simulink model "three_phase_pump"  (R2018a)
settings: Solver=VariableStepDiscrete  StartTime=0.0  StopTime=3  RelTol=1e-3
values from neighbouring files (symbols this model uses):
  Ts = 0.0001    [pump_ori_perf.mat]
libraries: fl_lib x8, sh_lib x5, nesl_utility x5, powerlib x2, electricdrivelib x1, powerlib_meascontrol x1
settings Model: Creator=siwak  LastModifiedBy=siwak

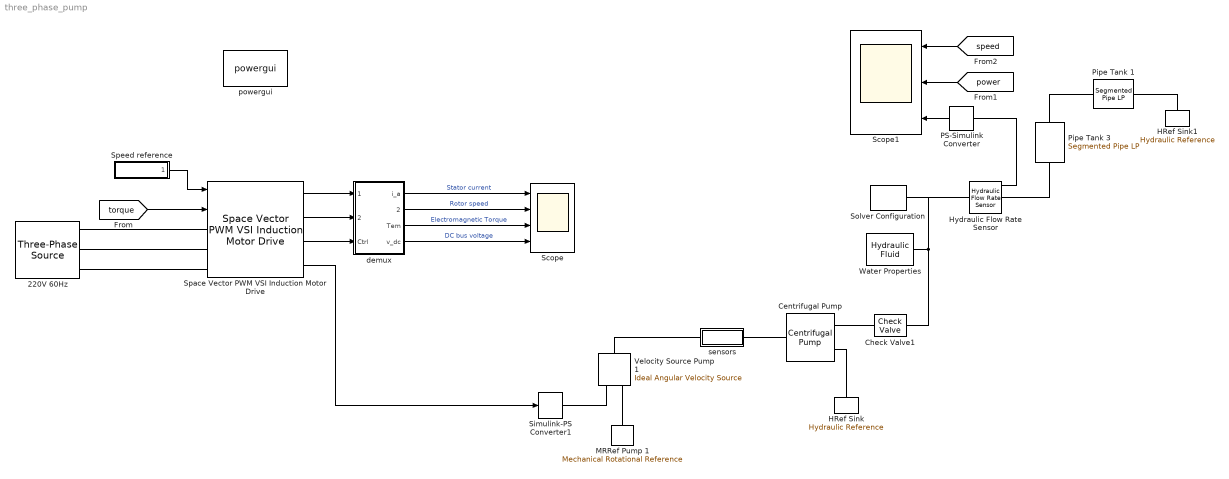
== system three_phase_pump ==
  220V 60Hz : powerlib/Electrical Sources/Three-Phase Source  InternalConnection=Yg  VoltagePhases=off  Voltage=220  PhaseAngle=0  Voltage_phases=[25e3 25e3 25e3]/sqrt(3)  PhaseAngles_phases=[0 -120 +120]  Frequency=60  NonIdealSource=on  SpecifyImpedance=off  Resistance=0.02  Inductance=0.05e-3  ShortCircuitLevel=100e6  BaseVoltage=25e3  XRratio=7  BusType=swing  Pref=0  Qref=0  Prefabc=[10e3, 10e3, 10e3]  Qrefabc=[0, 0, 0]  Qmin=-inf  Qmax=inf
  Centrifugal Pump : sh_lib/Pumps and Motors/Centrifugal Pump  mdl_type=2  c_1=326.8 Pa/(kg/m^3)  c_2=3.104e+4 Pa*s/kg  c_3=1.097e+7 Pa*s^2/(kg*m^3)  c_4=2.136e+5 Pa*s^2/(kg*m^3)  c_f=0.8  design_del=130 lpm  ref_velocity=1.77e+3 rpm  ref_density=940 kg/m^3  leak_resistance=1e+8 Pa/(m^3/s)  T_const=0.1 N*m  trq_press_coeff=1e-6 N*m/Pa  pump_del_1D="[ 0  20.0   64.2   92.8  110.0  130.0] gpm"  press_diff_1D=[50.97 47.08 39.12 31.39 23.6 15.69] psi  pump_del_power_1D="[ 0  20.0   64.2   92.8  110.0  130.0] gpm"  power_1D="[0 7.8e-01   2.1   2.4   2.16   1.7] HP"  pump_vel_2D=[ 3.2e+3 3.3e+3 3.4e+3 3.5e+3 ] rpm  pump_del_2D=[ 0 50 100 150 200 250 300 350 ] lpm  press_diff_2D=[ 8.3 8.8 9.3 9.9; 7.8 8.3 8.8 9.4; 7.2 7.6 8.2 8.7; 6.5 7 7.5 8; 5.6 6.1 6.6 7.1; 4.7 5.2 5.7 6.2; 3.4 4 4.4 4.9; 2.3 2.7 3.4 3.6 ] bar  pump_del_power_2D=[ 0 50 100 150 200 250 300 350 ] lpm  power_2D=[ 1.223e+3 1.341e+3 1.467e+3 1.6e+3; 1.414e+3 1.551e+3 1.696e+3 1.85e+3; 1.636e+3 1.794e+3 1.962e+3 2.14e+3; 1.941e+3 2.129e+3 2.326e+3 2.54e+3; 2.224e+3 2.439e+3 2.66e+3 2.91e+3; 2.453e+3 2.691e+3 2.947e+3 3.21e+3; 2.757e+3 3.024e+3 3.307e+3 3.608e+3; 2.945e+3 3.23e+3 3.533e+3 3.854e+3 ] W  omega_threshold=1e-9 rad/s  interp_method=3  extrap_method=1
      settings: SourceProductName=Simscape Fluids  SourceProductBaseCode=SH
  Check Valve1 : sh_lib/Valves/Directional Valves/Check Valve  area_max=3.8 in^2  pres_crack=0.8 psi  pres_max=2.5 psi  C_d=0.7  A_leak=1e-9 m^2  lam_spec=1  B_lam=0.999  Re_cr=12  dynamic=0  tau=0.1 s  area_init=1e-12 m^2
      settings: SourceProductName=Simscape Fluids  SourceProductBaseCode=SH
  HRef Sink : fl_lib/Hydraulic/Hydraulic Elements/Hydraulic Reference
      settings: SourceProductName=Simscape
  HRef Sink1 : fl_lib/Hydraulic/Hydraulic Elements/Hydraulic Reference
      settings: SourceProductName=Simscape
  Hydraulic Flow Rate Sensor : fl_lib/Hydraulic/Hydraulic Sensors/Hydraulic Flow Rate Sensor
      settings: SourceProductName=Simscape
  MRRef Pump 1 : fl_lib/Mechanical/Rotational Elements/Mechanical Rotational Reference
  PS-Simulink Converter : nesl_utility/PS-Simulink Converter  PhysicalDomain=network_engine_domain  SubClassName=ps_output  LeftPortType=input  RightPortType=output  PseudoPeriodic=off  Frequencies=[]  Unit=m^3/s  AffineConversion=off
  Pipe Tank 1 : sh_lib/Low-Pressure Blocks/Segmented Pipe LP  d_in=300 mm  length=850 m  segm_num=2  length_ad=406 m  roughness=1.5e-04 m  Re_lam=2e+03  Re_turb=4e+03  elevation_A=3 m  elevation_B=3 m  g=9.806649999999999 m/s^2  wall_type=1  pr_r_coef=2e-10 m/Pa  time_const=0.008 s  k_sh=1.4  p0_vec=0 Pa  q0=0 m^3/s
      settings: AttributesFormatString=%<elevation_A>%<elevation_A_unit> - %<elevation_B>%<elevation_B_unit>  SourceProductName=Simscape Fluids  SourceProductBaseCode=SH
  Pipe Tank 3 : sh_lib/Low-Pressure Blocks/Segmented Pipe LP  d_in=300 mm  length=850 m  segm_num=2  length_ad=406 m  roughness=1.5e-04 m  Re_lam=2e+03  Re_turb=4e+03  elevation_A=3 m  elevation_B=0.5 m  g=9.806649999999999 m/s^2  wall_type=1  pr_r_coef=2e-10 m/Pa  time_const=0.008 s  k_sh=1.4  p0_vec=0 Pa  q0=0 m^3/s
      settings: AttributesFormatString=%<elevation_A>%<elevation_A_unit> - %<elevation_B>%<elevation_B_unit>  SourceProductName=Simscape Fluids  SourceProductBaseCode=SH
  Scope : Scope  NumInputPorts=4
  Scope1 : Scope  NumInputPorts=3
  Simulink-PS Converter1 : nesl_utility/Simulink-PS Converter  PhysicalDomain=network_engine_domain  SubClassName=ps_input  LeftPortType=input  RightPortType=output  PseudoPeriodic=off  Frequencies=[]  NoiseDistribution=none  NoiseParameters=[]  Unit=rpm  AffineConversion=off  FilteringAndDerivatives=zero  SimscapeFilterOrder=1  InputFilterTimeConstant=.001  UdotUserProvided=0
  Solver Configuration : nesl_utility/Solver Configuration  PhysicalDomain=network_engine_domain  SubClassName=solver  LeftPortType=input  RightPortType=generic  Tones=[]  Harmonics=[]  SimulateNoise=off  Profile=off  UseLocalSampling=off  EnableSwitchedLinearOptims=on  FrequencyDomain=off  UseCCode=off  RelTol=0.001  AbsTol=1e-06  MinStep=1e-09  ToWorkspace=off  RevertToSquareIcSolve=off  NumHomotopyIterations=100  PhasorMode=off  PhasorModeNumHarmonics=1  DoDC=off  ResidualTolerance=1e-9  UseLocalSolver=on  LocalSolverChoice=NE_BACKWARD_EULER_ADVANCER  LocalSolverSampleTime=.01  DoFixedCost=on  MaxNonlinIter=3  MaxModeIter=2  LinearAlgebra=Sparse  EquationFormulation=NE_TIME_EF  DelaysMemoryBudget=1024  AutomaticFiltering=on  FilteringTimeConstant=0.001
  Space Vector PWM VSI Induction Motor Drive : electricdrivelib/AC drives/Space Vector PWM VSI Induction Motor Drive  ReferenceFrame=Stationary  IterativeDiscreteModel=Trapezoidal non iterative  Pn=2238  Vn=220  fn=60  Rs=0.435  Lls=0.002  Lms=69.31e-3  Rr=0.816  Llr=0.002  ia=0  pha=0  ib=0  phb=0  ic=0  phc=0  J=0.089  Friction=0.005  p=2  slip=1  thdeg=0  Rsnb_rec=10e3  Csnb_rec=20e-9  Ron_rec=1e-3  Vf_rec=1.3  cap_bus=3400e-6  Rbrake=8  fbrake=4000  activationVoltage=340  shutdownVoltage=320  deviceType=IGBT / Diodes  Ron_inv=1e-3  Vf_inv=1.2  Vfd_inv=1.2  Tf=1e-6  Tt=2e-6  Tf_GTO=10e-6  Tt_GTO=20e-6  Rsnb_inv=500  Csnb_inv=1e-9  Acc=1800  Dec=-1800  kp_sc=9  ki_sc=10  fc_sc=100  Tsc=100e-6  ctrl_sat_min=-30  ctrl_sat_max=30  ctrl_f_min=0.05  ctrl_f_max=120  ctrl_v_min=10  ctrl_v_max=180  vh_ratio=3.2  zc_time=0.4  car_freq=4500  fc_bus=50  Tvect=20e-6  baseSampleTime=2e-06  outputBusMode=Multiple output buses  busLabels=off  MechanicalLoad=Torque Tm  modelDetailLevel=Detailed  driveType=AC2  AverageValue=off
      settings: SourceProductName=Simscape Power Systems  SourceProductBaseCode=PS
  Speed reference : Subsystem
  Velocity Source Pump 1 : fl_lib/Mechanical/Mechanical Sources/Ideal Angular Velocity Source
  Water Properties : sh_lib/Hydraulic Utilities/Hydraulic Fluid  DataSource=1  SelFluid=24  SysTemp=1  TrapAir=0.001  ViscDerFactor=1  range_error=2
      settings: SourceProductName=Simscape Fluids
  demux : Subsystem
  powergui : powerlib/powergui  Priority=2  SimulationMode=Discrete  SampleTime=Ts  frequency=60  Iterations=50  frequencyindice=60  Pbase=100e6  ErrMax=1e-4  UnitsV=kV  UnitsW=MW  buscounter=0  FunctionMessages=off  echomessages=off  EnableUseOfTLC=off  CurrentSourceSwitches=off  DisableSnubberDevices=off  DisableRonSwitches=off  DisableVfSwitches=off  DisplayEquations=off  SolverType=Tustin/Backward Euler (TBE)  Interpol=off  ExternalGateDelay=off  methode=off  Ts=0  x0status=blocks  SPID=off  SwTol=0  HookPort=off  RestoreLinks=warning  ResistiveCurrentMeasurement=off  Frange=[0:2:500]  Ylog=off  Xlog=on  ShowGrid=off  save=off  variable=ZData  structure=0  ZoomFFT=on  StartTime=0.0  cycles=1  DisplayStyle=1  fundamental=60  FreqAxis=off  MaxFrequency=1000  frequencyindicesteady=1  RmsSteady=1  display=off
  sensors : Subsystem
  wires:
  demux/3(Tem) -> Scope/3  "Electromagnetic Torque"
  Space Vector PWM VSI Induction Motor Drive/2 -> demux/2(Conv.)
  Space Vector PWM VSI Induction Motor Drive/3 -> demux/3(Ctrl)
  Space Vector PWM VSI Induction Motor Drive/4 -> Simulink-PS Converter1/1
  Speed reference/1(" ") -> Space Vector PWM VSI Induction Motor Drive/1
  Space Vector PWM VSI Induction Motor Drive/1 -> demux/1(Motor)
  demux/2(speed) -> Scope/2  "Rotor speed"
  demux/4(v_dc) -> Scope/4  "DC bus voltage"
  demux/1(i_a) -> Scope/1  "Stator current"
  [torque] -> Space Vector PWM VSI Induction Motor Drive/2
  PS-Simulink Converter/1 -> Scope1/3
  [power] -> Scope1/2
  [speed] -> Scope1/1
  connections:
  220V 60Hz/RConn3 -- Space Vector PWM VSI Induction Motor Drive/LConn3
  220V 60Hz/RConn2 -- Space Vector PWM VSI Induction Motor Drive/LConn2
  220V 60Hz/RConn1 -- Space Vector PWM VSI Induction Motor Drive/LConn1
  Simulink-PS Converter1/RConn1 -- Velocity Source Pump 1/RConn1
  MRRef Pump 1/LConn1 -- Velocity Source Pump 1/RConn2
  sensors/LConn1 -- Velocity Source Pump 1/LConn1
  Centrifugal Pump/LConn1 -- sensors/RConn1
  Centrifugal Pump/RConn2 -- HRef Sink/LConn1
  Check Valve1/LConn1 -- Centrifugal Pump/RConn1
  Solver Configuration/RConn1 -- Hydraulic Flow Rate Sensor/LConn1 -- Check Valve1/RConn1 -- Water Properties/RConn1
  Pipe Tank 3/RConn1 -- Hydraulic Flow Rate Sensor/RConn2
  Pipe Tank 1/LConn1 -- Pipe Tank 3/LConn1
  Pipe Tank 1/RConn1 -- HRef Sink1/LConn1
  Hydraulic Flow Rate Sensor/RConn1 -- PS-Simulink Converter/LConn1

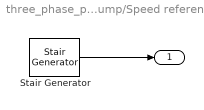
== system three_phase_pump/Speed reference ==
  Stair Generator : powerlib_meascontrol/Pulse & Signal Generators/Stair Generator  t=[1]  e=[1500]  Ts=Ts
      settings: SourceProductName=Simscape Power Systems
  " " : Outport
  wires:
  Stair Generator/1 -> " "/1

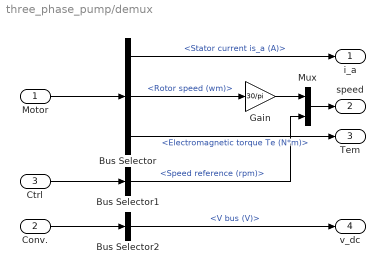
== system three_phase_pump/demux ==
  Motor : Inport
  Conv. : Inport  Port=2
  Ctrl : Inport  Port=3
  Bus Selector : BusSelector  OutputSignals=Stator measurements.Stator current is_a (A),Mechanical.Rotor speed (wm),Mechanical.Electromagnetic torque Te (N*m)
  Bus Selector1 : BusSelector  OutputSignals=Speed reference (rpm)
  Bus Selector2 : BusSelector  OutputSignals=V bus (V)
  Gain : Gain  Gain=30/pi  SaturateOnIntegerOverflow=on  OutDataTypeStr=Inherit: Same as input  ParamDataTypeStr=Inherit: Same as input
  Mux : Mux  Inputs=2
  i_a : Outport
  speed : Outport  Port=2
  Tem : Outport  Port=3
  v_dc : Outport  Port=4
  wires:
  Ctrl/1 -> Bus Selector1/1
  Gain/1 -> Mux/1
  Mux/1 -> speed/1
  Motor/1 -> Bus Selector/1
  Bus Selector/1 -> i_a/1  "<Stator current is_a (A)>"
  Bus Selector/2 -> Gain/1  "<Rotor speed (wm)>"
  Bus Selector/3 -> Tem/1  "<Electromagnetic torque Te (N*m)>"
  Bus Selector1/1 -> Mux/2  "<Speed reference (rpm)>"
  Conv./1 -> Bus Selector2/1
  Bus Selector2/1 -> v_dc/1  "<V bus (V)>"

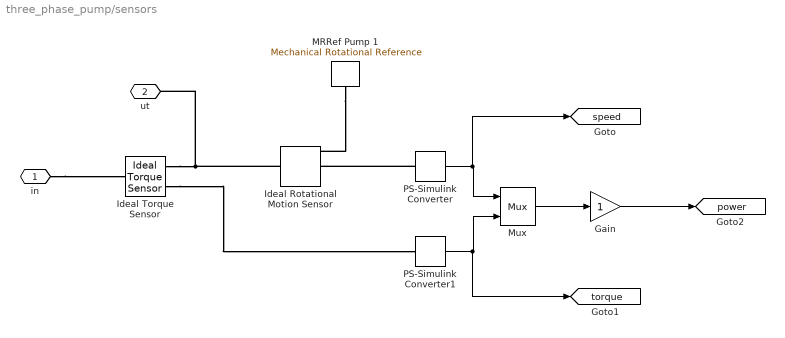
== system three_phase_pump/sensors ==
  Gain : Gain
  Ideal Rotational Motion Sensor : fl_lib/Mechanical/Mechanical Sensors/Ideal Rotational Motion Sensor  offset=0 rad
  Ideal Torque Sensor : fl_lib/Mechanical/Mechanical Sensors/Ideal Torque Sensor
  MRRef Pump 1 : fl_lib/Mechanical/Rotational Elements/Mechanical Rotational Reference
  Mux : Mux  Inputs=2
  PS-Simulink Converter : nesl_utility/PS-Simulink Converter  PhysicalDomain=network_engine_domain  SubClassName=ps_output  LeftPortType=input  RightPortType=output  PseudoPeriodic=off  Frequencies=[]  Unit=rad/s  AffineConversion=off
  PS-Simulink Converter1 : nesl_utility/PS-Simulink Converter  PhysicalDomain=network_engine_domain  SubClassName=ps_output  LeftPortType=input  RightPortType=output  PseudoPeriodic=off  Frequencies=[]  Unit=N*m  AffineConversion=off
  in : PMIOPort  Side=Left
  ut : PMIOPort  Port=2  Side=Right
  tag scope: power=global, speed=global, torque=global
  wires:
  PS-Simulink Converter/1 -> [speed], Mux/1
  PS-Simulink Converter1/1 -> [torque], Mux/2
  Mux/1 -> Gain/1
  Gain/1 -> [power]
  connections:
  in/RConn1 -- Ideal Torque Sensor/LConn1
  Ideal Torque Sensor/RConn1 -- Ideal Rotational Motion Sensor/LConn1 -- ut/RConn1
  MRRef Pump 1/LConn1 -- Ideal Rotational Motion Sensor/RConn1
  PS-Simulink Converter/LConn1 -- Ideal Rotational Motion Sensor/RConn2
  Ideal Torque Sensor/RConn2 -- PS-Simulink Converter1/LConn1
